simulink model "IEEE123bus_v2019b_Discrete_ZIPload"  (R2019b)
settings: Solver=ode4  StartTime=0.0  StopTime=5  FixedStep=Ts  MaxStep=1e-4  RelTol=1e-3
InitFcn:
  | a=1; % Loading Factor
  | Ts=50e-6;
  | % phase to sequence conversion of RXB matrices
  | c=1*exp(sqrt(-1)*(120*pi/180));
  | T=[1 1 1;1 c*c c;1 c c*c];
  | Tinv=1/3*[1 1 1;1 c c*c;1 c*c c];
  | 
  | % Simulation data for the IEEE 123 Node Test Feeder model
  | mi2km = 1.60934;%  miles to km conversion
  | ft2km = 0.0003048; % feet to km conversion
  | ms2F = 1*1e-6/(2*pi*60);% microsiemens to Farads conversion
  | 
  | %% Configuration 1
  | % Series Resitance and Reactance - ohm/mile
  | R_1 = [0.4576 0.1560 0.1535;0.1560 0.4666 0.1580;0.1535 0.1580 0.4615];
  | X_1 = [1.0780 0.5017 0.3849;0.5017 1.0482 0.4236;0.3849 0.4236 1.0651];
  | % charging susceptance - microsiemens/mile
  | B_1 = [5.6765 -1.8319 -0.6982;-1.8319 5.9809 -1.1645;-0.6982 -1.1645 5.3971];
  | 
  | R_1 = R_1/mi2km;
  | Rseq=Tinv*R_1*T;
  | R1_1=Rseq(2,2);R0_1=Rseq(1,1);
  | 
  | L_1 = (X_1/(2*pi*60))/mi2km;
  | Lseq=Tinv*L_1*T;
  | L1_1=Lseq(2,2);L0_1=Lseq(1,1);
  | 
  | C_1 =(B_1*ms2F)/mi2km;
  | Cseq=Tinv*C_1*T;
  | C1_1=Cseq(2,2);C0_1=Cseq(1,1);
  | %% Configuration 2 - series reactance - ohm/mile
  | R_2 = [0.4666 0.1580 0.1560;0.1580 0.4615 0.1535;0.1560 0.1535 0.4576];
  | X_2 = [1.0482 0.4236 0.5017;0.4236 1.0651 0.3849;0.5017 0.3849 1.0780];
  | % charging susceptance - microsiemens/mile
  | B_2 = [5.9809 -1.1645 -1.8319;-1.1645 5.3971 -0.6982;-1.8319 -0.6982 5.6765];
  | 
  | R_2 = R_2/mi2km;
  | Rseq=Tinv*R_2*T;
  | R1_2=Rseq(2,2);R0_2=Rseq(1,1);
  | 
  | L_2 = (X_2/(2*pi*60))/mi2km;
  | Lseq=Tinv*L_2*T;
  | L1_2=Lseq(2,2);L0_2=Lseq(1,1);
  | 
  | C_2 =(B_2*ms2F)/mi2km;
  | Cseq=Tinv*C_2*T;
  | C1_2=Cseq(2,2);C0_2=Cseq(1,1);
  | %% Configuration 3 - series reactance - ohm/mile
  | R_3 = [0.4615 0.1535 0.1580;0.1535 0.4576 0.1560;0.1580 0.1560 0.4666];
  | X_3 = [1.0651 0.3849 0.4236;0.3849 1.0780 0.5017;0.4236 0.5017 1.0482];
  | % charging susceptance - microsiemens/mile
  | B_3 = [5.3971 -0.6982 -1.1645;-0.6982 5.6765 -1.8319; -1.1645 -1.8319 5.9809];
  | 
  | R_3 = R_3/mi2km;
  | Rseq=Tinv*R_3*T;
  | R1_3=Rseq(2,2);R0_3=Rseq(1,1);
  | 
  | L_3 = (X_3/(2*pi*60))/mi2km;
  | Lseq=Tinv*L_3*T;
  | L1_3=Lseq(2,2);L0_3=Lseq(1,1);
  | ... (+157 lines)
undefined symbols (not defined in the file): D1, Delta, find_system
libraries: powerlib x971, powerlib_meascontrol x294
(part 3 of 14)

== system IEEE123bus_v2019b_Discrete_ZIPload/1 Y PQ ==
  "    1" : Gain  Gain=pi/180
  "    2" : Gain  Gain=pi/180
  "    3" : Gain  Gain=pi/180
  "    4" : Gain  Gain=1/sqrt(2)
  Clock : Clock
  Controlled Current Source : powerlib/Electrical Sources/Controlled Current Source  Initialize=off  Source_Type=AC  Amplitude=0  Phase=0  Frequency=0  Measurements=None
      settings: SourceProductName=Simscape Electrical
  Embedded MATLAB Function : MATLAB Function  TreatAsAtomicUnit=on
  Fourier : powerlib_meascontrol/Measurements/Fourier  Freq=60  n=1  InInit=[Vnom*sqrt(2) 0]  Ts=Ts
      settings: SourceProductName=Simscape Electrical
  Fourier1 : powerlib_meascontrol/Measurements/Fourier  Freq=60  n=1  InInit=[Vnom*sqrt(2) 0]  Ts=Ts
      settings: SourceProductName=Simscape Electrical
  Fourier2 : powerlib_meascontrol/Measurements/Fourier  Freq=60  n=1  InInit=[Vnom*sqrt(2) 0]  Ts=Ts
      settings: SourceProductName=Simscape Electrical
  Magnitude-Angle to Complex : MagnitudeAngleToComplex
  Memory1 : Memory
  Memory2 : Memory
  Rc+jXc1 : powerlib/Elements/Series RLC Branch  LConnTagsString=__new0  RConnTagsString=__new0  BranchType=R  Resistance=1e6  Inductance=1.6 / (120*pi) * 2  SetiL0=off  InitialCurrent=0  Capacitance=1e-6  Setx0=off  InitialVoltage=0  Measurements=None
      settings: SourceProductName=Simscape Electrical
  Sum : Sum  Inputs=|+-
  Voltage Measurement1 : powerlib/Measurements/Voltage Measurement  PhasorSimulation=off  OutputType=Complex  PSBequivalent=0
      settings: SourceProductName=Simscape Electrical
  " " : PMIOPort  Tag=PMCPort  Side=Left
  " 1" : PMIOPort  Tag=PMCPort  Port=2  Side=Right
  wires:
  Fourier/2 -> "    3"/1
  "    1"/1 -> Sum/1
  Voltage Measurement1/1 -> [v]
  [del] -> Embedded MATLAB Function/3(Ddel)
  Memory2/1 -> [del]
  Sum/1 -> Memory2/1
  "    2"/1 -> Sum/2
  [v] -> Fourier/1
  Fourier/1 -> "    4"/1
  Embedded MATLAB Function/1(Iinjinst) -> Memory1/1, Fourier1/1
  Fourier1/2 -> "    1"/1
  Memory1/1 -> Controlled Current Source/1, Fourier2/1
  Clock/1 -> Embedded MATLAB Function/2(clock)
  Magnitude-Angle to Complex/1 -> Embedded MATLAB Function/1(Vmeas)
  "    4"/1 -> Magnitude-Angle to Complex/1
  Fourier2/2 -> "    2"/1
  "    3"/1 -> Magnitude-Angle to Complex/2
  connections:
  Rc+jXc1/LConn1 -- Voltage Measurement1/LConn1 -- " "/RConn1 -- Controlled Current Source/LConn1
  Voltage Measurement1/LConn2 -- " 1"/RConn1 -- Controlled Current Source/RConn1 -- Rc+jXc1/RConn1

== system IEEE123bus_v2019b_Discrete_ZIPload/10 ==
  2 : powerlib/Measurements/Three-Phase V-I Measurement  VoltageMeasurement=phase-to-ground  SetLabelV=on  LabelV=V10  Vpu=off  VpuLL=off  CurrentMeasurement=no  SetLabelI=on  LabelI=I800  Ipu=off  Pbase=100e6  Vbase=24900  OutputType=Complex  PhasorSimulation=on  PSBequivalent=0
      settings: SourceProductName=Simscape Electrical
  Ground82 : powerlib/Elements/Ground  LConnTagsString=a
      settings: SourceProductName=Simscape Electrical
  Ground83 : powerlib/Elements/Ground  LConnTagsString=a
      settings: SourceProductName=Simscape Electrical
  a : PMIOPort  Side=Right
  A : PMIOPort  Port=2  Side=Left
  connections:
  A/RConn1 -- 2/LConn1
  a/RConn1 -- 2/RConn1
  2/LConn2 -- 2/LConn3 -- Ground83/LConn1
  2/RConn2 -- 2/RConn3 -- Ground82/LConn1

== system IEEE123bus_v2019b_Discrete_ZIPload/10 Y I ==
  "    1" : Gain  Gain=pi/180
  "    2" : Gain  Gain=pi/180
  "    3" : Gain  Gain=pi/180
  "    4" : Gain  Gain=1/sqrt(2)
  Clock : Clock
  Controlled Current Source : powerlib/Electrical Sources/Controlled Current Source  Initialize=off  Source_Type=AC  Amplitude=0  Phase=0  Frequency=0  Measurements=None
      settings: SourceProductName=Simscape Electrical
  Embedded MATLAB Function : MATLAB Function  TreatAsAtomicUnit=on
  Fourier : powerlib_meascontrol/Measurements/Fourier  Freq=60  n=1  InInit=[Vnom*sqrt(2) 0]  Ts=Ts
      settings: SourceProductName=Simscape Electrical
  Fourier1 : powerlib_meascontrol/Measurements/Fourier  Freq=60  n=1  InInit=[Vnom*sqrt(2) 0]  Ts=Ts
      settings: SourceProductName=Simscape Electrical
  Fourier2 : powerlib_meascontrol/Measurements/Fourier  Freq=60  n=1  InInit=[Vnom*sqrt(2) 0]  Ts=Ts
      settings: SourceProductName=Simscape Electrical
  Magnitude-Angle to Complex : MagnitudeAngleToComplex
  Memory1 : Memory
  Memory2 : Memory
  Rc+jXc1 : powerlib/Elements/Series RLC Branch  LConnTagsString=__new0  RConnTagsString=__new0  BranchType=R  Resistance=1e6  Inductance=1.6 / (120*pi) * 2  SetiL0=off  InitialCurrent=0  Capacitance=1e-6  Setx0=off  InitialVoltage=0  Measurements=None
      settings: SourceProductName=Simscape Electrical
  Sum : Sum  Inputs=|+-
  Voltage Measurement1 : powerlib/Measurements/Voltage Measurement  PhasorSimulation=off  OutputType=Complex  PSBequivalent=0
      settings: SourceProductName=Simscape Electrical
  " " : PMIOPort  Tag=PMCPort  Side=Left
  " 1" : PMIOPort  Tag=PMCPort  Port=2  Side=Right
  wires:
  Fourier/2 -> "    3"/1
  "    1"/1 -> Sum/1
  Voltage Measurement1/1 -> [v]
  [del] -> Embedded MATLAB Function/3(Ddel)
  Memory2/1 -> [del]
  Sum/1 -> Memory2/1
  "    2"/1 -> Sum/2
  [v] -> Fourier/1
  Fourier/1 -> "    4"/1
  Embedded MATLAB Function/1(Iinjinst) -> Memory1/1, Fourier1/1
  Fourier1/2 -> "    1"/1
  Memory1/1 -> Controlled Current Source/1, Fourier2/1
  Clock/1 -> Embedded MATLAB Function/2(clock)
  Magnitude-Angle to Complex/1 -> Embedded MATLAB Function/1(Vmeas)
  "    4"/1 -> Magnitude-Angle to Complex/1
  Fourier2/2 -> "    2"/1
  "    3"/1 -> Magnitude-Angle to Complex/2
  connections:
  Rc+jXc1/LConn1 -- Voltage Measurement1/LConn1 -- " "/RConn1 -- Controlled Current Source/LConn1
  Voltage Measurement1/LConn2 -- " 1"/RConn1 -- Controlled Current Source/RConn1 -- Rc+jXc1/RConn1

== system IEEE123bus_v2019b_Discrete_ZIPload/100 Y Z ==
  "    1" : Gain  Gain=pi/180
  "    2" : Gain  Gain=pi/180
  "    3" : Gain  Gain=pi/180
  "    4" : Gain  Gain=1/sqrt(2)
  Clock : Clock
  Controlled Current Source : powerlib/Electrical Sources/Controlled Current Source  Initialize=off  Source_Type=AC  Amplitude=0  Phase=0  Frequency=0  Measurements=None
      settings: SourceProductName=Simscape Electrical
  Embedded MATLAB Function : MATLAB Function  TreatAsAtomicUnit=on
  Fourier : powerlib_meascontrol/Measurements/Fourier  Freq=60  n=1  InInit=[Vnom*sqrt(2) 0]  Ts=Ts
      settings: SourceProductName=Simscape Electrical
  Fourier1 : powerlib_meascontrol/Measurements/Fourier  Freq=60  n=1  InInit=[Vnom*sqrt(2) 0]  Ts=Ts
      settings: SourceProductName=Simscape Electrical
  Fourier2 : powerlib_meascontrol/Measurements/Fourier  Freq=60  n=1  InInit=[Vnom*sqrt(2) 0]  Ts=Ts
      settings: SourceProductName=Simscape Electrical
  Magnitude-Angle to Complex : MagnitudeAngleToComplex
  Memory1 : Memory
  Memory2 : Memory
  Rc+jXc1 : powerlib/Elements/Series RLC Branch  LConnTagsString=__new0  RConnTagsString=__new0  BranchType=R  Resistance=1e6  Inductance=1.6 / (120*pi) * 2  SetiL0=off  InitialCurrent=0  Capacitance=1e-6  Setx0=off  InitialVoltage=0  Measurements=None
      settings: SourceProductName=Simscape Electrical
  Sum : Sum  Inputs=|+-
  Voltage Measurement1 : powerlib/Measurements/Voltage Measurement  PhasorSimulation=off  OutputType=Complex  PSBequivalent=0
      settings: SourceProductName=Simscape Electrical
  " " : PMIOPort  Tag=PMCPort  Side=Left
  " 1" : PMIOPort  Tag=PMCPort  Port=2  Side=Right
  wires:
  Fourier/2 -> "    3"/1
  "    1"/1 -> Sum/1
  Voltage Measurement1/1 -> [v]
  [del] -> Embedded MATLAB Function/3(Ddel)
  Memory2/1 -> [del]
  Sum/1 -> Memory2/1
  "    2"/1 -> Sum/2
  [v] -> Fourier/1
  Fourier/1 -> "    4"/1
  Embedded MATLAB Function/1(Iinjinst) -> Memory1/1, Fourier1/1
  Fourier1/2 -> "    1"/1
  Memory1/1 -> Controlled Current Source/1, Fourier2/1
  Clock/1 -> Embedded MATLAB Function/2(clock)
  Magnitude-Angle to Complex/1 -> Embedded MATLAB Function/1(Vmeas)
  "    4"/1 -> Magnitude-Angle to Complex/1
  Fourier2/2 -> "    2"/1
  "    3"/1 -> Magnitude-Angle to Complex/2
  connections:
  Rc+jXc1/LConn1 -- Voltage Measurement1/LConn1 -- " "/RConn1 -- Controlled Current Source/LConn1
  Voltage Measurement1/LConn2 -- " 1"/RConn1 -- Controlled Current Source/RConn1 -- Rc+jXc1/RConn1

== system IEEE123bus_v2019b_Discrete_ZIPload/102 ==
  2 : powerlib/Measurements/Three-Phase V-I Measurement  VoltageMeasurement=phase-to-ground  SetLabelV=on  LabelV=V102  Vpu=off  VpuLL=off  CurrentMeasurement=no  SetLabelI=on  LabelI=I800  Ipu=off  Pbase=100e6  Vbase=24900  OutputType=Complex  PhasorSimulation=on  PSBequivalent=0
      settings: SourceProductName=Simscape Electrical
  Ground82 : powerlib/Elements/Ground  LConnTagsString=a
      settings: SourceProductName=Simscape Electrical
  Ground83 : powerlib/Elements/Ground  LConnTagsString=a
      settings: SourceProductName=Simscape Electrical
  c : PMIOPort  Side=Right
  C : PMIOPort  Port=2  Side=Left
  connections:
  C/RConn1 -- 2/LConn3
  c/RConn1 -- 2/RConn3
  Ground82/LConn1 -- 2/RConn2 -- 2/RConn1
  Ground83/LConn1 -- 2/LConn2 -- 2/LConn1

== system IEEE123bus_v2019b_Discrete_ZIPload/102 Y PQ ==
  "    1" : Gain  Gain=pi/180
  "    2" : Gain  Gain=pi/180
  "    3" : Gain  Gain=pi/180
  "    4" : Gain  Gain=1/sqrt(2)
  Clock : Clock
  Controlled Current Source : powerlib/Electrical Sources/Controlled Current Source  Initialize=off  Source_Type=AC  Amplitude=0  Phase=0  Frequency=0  Measurements=None
      settings: SourceProductName=Simscape Electrical
  Embedded MATLAB Function : MATLAB Function  TreatAsAtomicUnit=on
  Fourier : powerlib_meascontrol/Measurements/Fourier  Freq=60  n=1  InInit=[Vnom*sqrt(2) 0]  Ts=Ts
      settings: SourceProductName=Simscape Electrical
  Fourier1 : powerlib_meascontrol/Measurements/Fourier  Freq=60  n=1  InInit=[Vnom*sqrt(2) 0]  Ts=Ts
      settings: SourceProductName=Simscape Electrical
  Fourier2 : powerlib_meascontrol/Measurements/Fourier  Freq=60  n=1  InInit=[Vnom*sqrt(2) 0]  Ts=Ts
      settings: SourceProductName=Simscape Electrical
  Magnitude-Angle to Complex : MagnitudeAngleToComplex
  Memory1 : Memory
  Memory2 : Memory
  Rc+jXc1 : powerlib/Elements/Series RLC Branch  LConnTagsString=__new0  RConnTagsString=__new0  BranchType=R  Resistance=1e6  Inductance=1.6 / (120*pi) * 2  SetiL0=off  InitialCurrent=0  Capacitance=1e-6  Setx0=off  InitialVoltage=0  Measurements=None
      settings: SourceProductName=Simscape Electrical
  Sum : Sum  Inputs=|+-
  Voltage Measurement1 : powerlib/Measurements/Voltage Measurement  PhasorSimulation=off  OutputType=Complex  PSBequivalent=0
      settings: SourceProductName=Simscape Electrical
  " " : PMIOPort  Tag=PMCPort  Side=Left
  " 1" : PMIOPort  Tag=PMCPort  Port=2  Side=Right
  wires:
  Fourier/2 -> "    3"/1
  "    1"/1 -> Sum/1
  Voltage Measurement1/1 -> [v]
  [del] -> Embedded MATLAB Function/3(Ddel)
  Memory2/1 -> [del]
  Sum/1 -> Memory2/1
  "    2"/1 -> Sum/2
  [v] -> Fourier/1
  Fourier/1 -> "    4"/1
  Embedded MATLAB Function/1(Iinjinst) -> Memory1/1, Fourier1/1
  Fourier1/2 -> "    1"/1
  Memory1/1 -> Controlled Current Source/1, Fourier2/1
  Clock/1 -> Embedded MATLAB Function/2(clock)
  Magnitude-Angle to Complex/1 -> Embedded MATLAB Function/1(Vmeas)
  "    4"/1 -> Magnitude-Angle to Complex/1
  Fourier2/2 -> "    2"/1
  "    3"/1 -> Magnitude-Angle to Complex/2
  connections:
  Rc+jXc1/LConn1 -- Voltage Measurement1/LConn1 -- " "/RConn1 -- Controlled Current Source/LConn1
  Voltage Measurement1/LConn2 -- " 1"/RConn1 -- Controlled Current Source/RConn1 -- Rc+jXc1/RConn1

== system IEEE123bus_v2019b_Discrete_ZIPload/103 ==
  2 : powerlib/Measurements/Three-Phase V-I Measurement  VoltageMeasurement=phase-to-ground  SetLabelV=on  LabelV=V103  Vpu=off  VpuLL=off  CurrentMeasurement=no  SetLabelI=on  LabelI=I800  Ipu=off  Pbase=100e6  Vbase=24900  OutputType=Complex  PhasorSimulation=on  PSBequivalent=0
      settings: SourceProductName=Simscape Electrical
  Ground82 : powerlib/Elements/Ground  LConnTagsString=a
      settings: SourceProductName=Simscape Electrical
  Ground83 : powerlib/Elements/Ground  LConnTagsString=a
      settings: SourceProductName=Simscape Electrical
  c : PMIOPort  Side=Right
  C : PMIOPort  Port=2  Side=Left
  connections:
  2/LConn1 -- 2/LConn2 -- Ground83/LConn1
  2/RConn1 -- 2/RConn2 -- Ground82/LConn1
  c/RConn1 -- 2/RConn3
  C/RConn1 -- 2/LConn3

== system IEEE123bus_v2019b_Discrete_ZIPload/103 Y PQ ==
  "    1" : Gain  Gain=pi/180
  "    2" : Gain  Gain=pi/180
  "    3" : Gain  Gain=pi/180
  "    4" : Gain  Gain=1/sqrt(2)
  Clock : Clock
  Controlled Current Source : powerlib/Electrical Sources/Controlled Current Source  Initialize=off  Source_Type=AC  Amplitude=0  Phase=0  Frequency=0  Measurements=None
      settings: SourceProductName=Simscape Electrical
  Embedded MATLAB Function : MATLAB Function  TreatAsAtomicUnit=on
  Fourier : powerlib_meascontrol/Measurements/Fourier  Freq=60  n=1  InInit=[Vnom*sqrt(2) 0]  Ts=Ts
      settings: SourceProductName=Simscape Electrical
  Fourier1 : powerlib_meascontrol/Measurements/Fourier  Freq=60  n=1  InInit=[Vnom*sqrt(2) 0]  Ts=Ts
      settings: SourceProductName=Simscape Electrical
  Fourier2 : powerlib_meascontrol/Measurements/Fourier  Freq=60  n=1  InInit=[Vnom*sqrt(2) 0]  Ts=Ts
      settings: SourceProductName=Simscape Electrical
  Magnitude-Angle to Complex : MagnitudeAngleToComplex
  Memory1 : Memory
  Memory2 : Memory
  Rc+jXc1 : powerlib/Elements/Series RLC Branch  LConnTagsString=__new0  RConnTagsString=__new0  BranchType=R  Resistance=1e6  Inductance=1.6 / (120*pi) * 2  SetiL0=off  InitialCurrent=0  Capacitance=1e-6  Setx0=off  InitialVoltage=0  Measurements=None
      settings: SourceProductName=Simscape Electrical
  Sum : Sum  Inputs=|+-
  Voltage Measurement1 : powerlib/Measurements/Voltage Measurement  PhasorSimulation=off  OutputType=Complex  PSBequivalent=0
      settings: SourceProductName=Simscape Electrical
  " " : PMIOPort  Tag=PMCPort  Side=Left
  " 1" : PMIOPort  Tag=PMCPort  Port=2  Side=Right
  wires:
  Fourier/2 -> "    3"/1
  "    1"/1 -> Sum/1
  Voltage Measurement1/1 -> [v]
  [del] -> Embedded MATLAB Function/3(Ddel)
  Memory2/1 -> [del]
  Sum/1 -> Memory2/1
  "    2"/1 -> Sum/2
  [v] -> Fourier/1
  Fourier/1 -> "    4"/1
  Embedded MATLAB Function/1(Iinjinst) -> Memory1/1, Fourier1/1
  Fourier1/2 -> "    1"/1
  Memory1/1 -> Controlled Current Source/1, Fourier2/1
  Clock/1 -> Embedded MATLAB Function/2(clock)
  Magnitude-Angle to Complex/1 -> Embedded MATLAB Function/1(Vmeas)
  "    4"/1 -> Magnitude-Angle to Complex/1
  Fourier2/2 -> "    2"/1
  "    3"/1 -> Magnitude-Angle to Complex/2
  connections:
  Rc+jXc1/LConn1 -- Voltage Measurement1/LConn1 -- " "/RConn1 -- Controlled Current Source/LConn1
  Voltage Measurement1/LConn2 -- " 1"/RConn1 -- Controlled Current Source/RConn1 -- Rc+jXc1/RConn1

== system IEEE123bus_v2019b_Discrete_ZIPload/104 ==
  2 : powerlib/Measurements/Three-Phase V-I Measurement  VoltageMeasurement=phase-to-ground  SetLabelV=on  LabelV=V104  Vpu=off  VpuLL=off  CurrentMeasurement=no  SetLabelI=on  LabelI=I800  Ipu=off  Pbase=100e6  Vbase=24900  OutputType=Complex  PhasorSimulation=on  PSBequivalent=0
      settings: SourceProductName=Simscape Electrical
  Ground82 : powerlib/Elements/Ground  LConnTagsString=a
      settings: SourceProductName=Simscape Electrical
  Ground83 : powerlib/Elements/Ground  LConnTagsString=a
      settings: SourceProductName=Simscape Electrical
  c : PMIOPort  Side=Right
  C : PMIOPort  Port=2  Side=Left
  connections:
  C/RConn1 -- 2/LConn3
  c/RConn1 -- 2/RConn3
  Ground82/LConn1 -- 2/RConn2 -- 2/RConn1
  Ground83/LConn1 -- 2/LConn2 -- 2/LConn1

== system IEEE123bus_v2019b_Discrete_ZIPload/104 Y PQ ==
  "    1" : Gain  Gain=pi/180
  "    2" : Gain  Gain=pi/180
  "    3" : Gain  Gain=pi/180
  "    4" : Gain  Gain=1/sqrt(2)
  Clock : Clock
  Controlled Current Source : powerlib/Electrical Sources/Controlled Current Source  Initialize=off  Source_Type=AC  Amplitude=0  Phase=0  Frequency=0  Measurements=None
      settings: SourceProductName=Simscape Electrical
  Embedded MATLAB Function : MATLAB Function  TreatAsAtomicUnit=on
  Fourier : powerlib_meascontrol/Measurements/Fourier  Freq=60  n=1  InInit=[Vnom*sqrt(2) 0]  Ts=Ts
      settings: SourceProductName=Simscape Electrical
  Fourier1 : powerlib_meascontrol/Measurements/Fourier  Freq=60  n=1  InInit=[Vnom*sqrt(2) 0]  Ts=Ts
      settings: SourceProductName=Simscape Electrical
  Fourier2 : powerlib_meascontrol/Measurements/Fourier  Freq=60  n=1  InInit=[Vnom*sqrt(2) 0]  Ts=Ts
      settings: SourceProductName=Simscape Electrical
  Magnitude-Angle to Complex : MagnitudeAngleToComplex
  Memory1 : Memory
  Memory2 : Memory
  Rc+jXc1 : powerlib/Elements/Series RLC Branch  LConnTagsString=__new0  RConnTagsString=__new0  BranchType=R  Resistance=1e6  Inductance=1.6 / (120*pi) * 2  SetiL0=off  InitialCurrent=0  Capacitance=1e-6  Setx0=off  InitialVoltage=0  Measurements=None
      settings: SourceProductName=Simscape Electrical
  Sum : Sum  Inputs=|+-
  Voltage Measurement1 : powerlib/Measurements/Voltage Measurement  PhasorSimulation=off  OutputType=Complex  PSBequivalent=0
      settings: SourceProductName=Simscape Electrical
  " " : PMIOPort  Tag=PMCPort  Side=Left
  " 1" : PMIOPort  Tag=PMCPort  Port=2  Side=Right
  wires:
  Fourier/2 -> "    3"/1
  "    1"/1 -> Sum/1
  Voltage Measurement1/1 -> [v]
  [del] -> Embedded MATLAB Function/3(Ddel)
  Memory2/1 -> [del]
  Sum/1 -> Memory2/1
  "    2"/1 -> Sum/2
  [v] -> Fourier/1
  Fourier/1 -> "    4"/1
  Embedded MATLAB Function/1(Iinjinst) -> Memory1/1, Fourier1/1
  Fourier1/2 -> "    1"/1
  Memory1/1 -> Controlled Current Source/1, Fourier2/1
  Clock/1 -> Embedded MATLAB Function/2(clock)
  Magnitude-Angle to Complex/1 -> Embedded MATLAB Function/1(Vmeas)
  "    4"/1 -> Magnitude-Angle to Complex/1
  Fourier2/2 -> "    2"/1
  "    3"/1 -> Magnitude-Angle to Complex/2
  connections:
  Rc+jXc1/LConn1 -- Voltage Measurement1/LConn1 -- " "/RConn1 -- Controlled Current Source/LConn1
  Voltage Measurement1/LConn2 -- " 1"/RConn1 -- Controlled Current Source/RConn1 -- Rc+jXc1/RConn1

== system IEEE123bus_v2019b_Discrete_ZIPload/106 ==
  2 : powerlib/Measurements/Three-Phase V-I Measurement  VoltageMeasurement=phase-to-ground  SetLabelV=on  LabelV=V106  Vpu=off  VpuLL=off  CurrentMeasurement=no  SetLabelI=on  LabelI=I800  Ipu=off  Pbase=100e6  Vbase=24900  OutputType=Complex  PhasorSimulation=on  PSBequivalent=0
      settings: SourceProductName=Simscape Electrical
  Ground82 : powerlib/Elements/Ground  LConnTagsString=a
      settings: SourceProductName=Simscape Electrical
  Ground83 : powerlib/Elements/Ground  LConnTagsString=a
      settings: SourceProductName=Simscape Electrical
  b : PMIOPort  Side=Right
  B : PMIOPort  Port=2  Side=Left
  connections:
  Ground82/LConn1 -- 2/RConn3 -- 2/RConn1
  Ground83/LConn1 -- 2/LConn3 -- 2/LConn1
  2/RConn2 -- b/RConn1
  2/LConn2 -- B/RConn1

== system IEEE123bus_v2019b_Discrete_ZIPload/106 Y PQ ==
  "    1" : Gain  Gain=pi/180
  "    2" : Gain  Gain=pi/180
  "    3" : Gain  Gain=pi/180
  "    4" : Gain  Gain=1/sqrt(2)
  Clock : Clock
  Controlled Current Source : powerlib/Electrical Sources/Controlled Current Source  Initialize=off  Source_Type=AC  Amplitude=0  Phase=0  Frequency=0  Measurements=None
      settings: SourceProductName=Simscape Electrical
  Embedded MATLAB Function : MATLAB Function  TreatAsAtomicUnit=on
  Fourier : powerlib_meascontrol/Measurements/Fourier  Freq=60  n=1  InInit=[Vnom*sqrt(2) 0]  Ts=Ts
      settings: SourceProductName=Simscape Electrical
  Fourier1 : powerlib_meascontrol/Measurements/Fourier  Freq=60  n=1  InInit=[Vnom*sqrt(2) 0]  Ts=Ts
      settings: SourceProductName=Simscape Electrical
  Fourier2 : powerlib_meascontrol/Measurements/Fourier  Freq=60  n=1  InInit=[Vnom*sqrt(2) 0]  Ts=Ts
      settings: SourceProductName=Simscape Electrical
  Magnitude-Angle to Complex : MagnitudeAngleToComplex
  Memory1 : Memory
  Memory2 : Memory
  Rc+jXc1 : powerlib/Elements/Series RLC Branch  LConnTagsString=__new0  RConnTagsString=__new0  BranchType=R  Resistance=1e6  Inductance=1.6 / (120*pi) * 2  SetiL0=off  InitialCurrent=0  Capacitance=1e-6  Setx0=off  InitialVoltage=0  Measurements=None
      settings: SourceProductName=Simscape Electrical
  Sum : Sum  Inputs=|+-
  Voltage Measurement1 : powerlib/Measurements/Voltage Measurement  PhasorSimulation=off  OutputType=Complex  PSBequivalent=0
      settings: SourceProductName=Simscape Electrical
  " " : PMIOPort  Tag=PMCPort  Side=Left
  " 1" : PMIOPort  Tag=PMCPort  Port=2  Side=Right
  wires:
  Fourier/2 -> "    3"/1
  "    1"/1 -> Sum/1
  Voltage Measurement1/1 -> [v]
  [del] -> Embedded MATLAB Function/3(Ddel)
  Memory2/1 -> [del]
  Sum/1 -> Memory2/1
  "    2"/1 -> Sum/2
  [v] -> Fourier/1
  Fourier/1 -> "    4"/1
  Embedded MATLAB Function/1(Iinjinst) -> Memory1/1, Fourier1/1
  Fourier1/2 -> "    1"/1
  Memory1/1 -> Controlled Current Source/1, Fourier2/1
  Clock/1 -> Embedded MATLAB Function/2(clock)
  Magnitude-Angle to Complex/1 -> Embedded MATLAB Function/1(Vmeas)
  "    4"/1 -> Magnitude-Angle to Complex/1
  Fourier2/2 -> "    2"/1
  "    3"/1 -> Magnitude-Angle to Complex/2
  connections:
  Rc+jXc1/LConn1 -- Voltage Measurement1/LConn1 -- " "/RConn1 -- Controlled Current Source/LConn1
  Voltage Measurement1/LConn2 -- " 1"/RConn1 -- Controlled Current Source/RConn1 -- Rc+jXc1/RConn1

== system IEEE123bus_v2019b_Discrete_ZIPload/107 ==
  2 : powerlib/Measurements/Three-Phase V-I Measurement  VoltageMeasurement=phase-to-ground  SetLabelV=on  LabelV=V107  Vpu=off  VpuLL=off  CurrentMeasurement=no  SetLabelI=on  LabelI=I800  Ipu=off  Pbase=100e6  Vbase=24900  OutputType=Complex  PhasorSimulation=on  PSBequivalent=0
      settings: SourceProductName=Simscape Electrical
  Ground82 : powerlib/Elements/Ground  LConnTagsString=a
      settings: SourceProductName=Simscape Electrical
  Ground83 : powerlib/Elements/Ground  LConnTagsString=a
      settings: SourceProductName=Simscape Electrical
  b : PMIOPort  Side=Right
  B : PMIOPort  Port=2  Side=Left
  connections:
  2/LConn2 -- B/RConn1
  2/RConn2 -- b/RConn1
  2/LConn1 -- 2/LConn3 -- Ground83/LConn1
  2/RConn1 -- 2/RConn3 -- Ground82/LConn1

== system IEEE123bus_v2019b_Discrete_ZIPload/107 Y PQ ==
  "    1" : Gain  Gain=pi/180
  "    2" : Gain  Gain=pi/180
  "    3" : Gain  Gain=pi/180
  "    4" : Gain  Gain=1/sqrt(2)
  Clock : Clock
  Controlled Current Source : powerlib/Electrical Sources/Controlled Current Source  Initialize=off  Source_Type=AC  Amplitude=0  Phase=0  Frequency=0  Measurements=None
      settings: SourceProductName=Simscape Electrical
  Embedded MATLAB Function : MATLAB Function  TreatAsAtomicUnit=on
  Fourier : powerlib_meascontrol/Measurements/Fourier  Freq=60  n=1  InInit=[Vnom*sqrt(2) 0]  Ts=Ts
      settings: SourceProductName=Simscape Electrical
  Fourier1 : powerlib_meascontrol/Measurements/Fourier  Freq=60  n=1  InInit=[Vnom*sqrt(2) 0]  Ts=Ts
      settings: SourceProductName=Simscape Electrical
  Fourier2 : powerlib_meascontrol/Measurements/Fourier  Freq=60  n=1  InInit=[Vnom*sqrt(2) 0]  Ts=Ts
      settings: SourceProductName=Simscape Electrical
  Magnitude-Angle to Complex : MagnitudeAngleToComplex
  Memory1 : Memory
  Memory2 : Memory
  Rc+jXc1 : powerlib/Elements/Series RLC Branch  LConnTagsString=__new0  RConnTagsString=__new0  BranchType=R  Resistance=1e6  Inductance=1.6 / (120*pi) * 2  SetiL0=off  InitialCurrent=0  Capacitance=1e-6  Setx0=off  InitialVoltage=0  Measurements=None
      settings: SourceProductName=Simscape Electrical
  Sum : Sum  Inputs=|+-
  Voltage Measurement1 : powerlib/Measurements/Voltage Measurement  PhasorSimulation=off  OutputType=Complex  PSBequivalent=0
      settings: SourceProductName=Simscape Electrical
  " " : PMIOPort  Tag=PMCPort  Side=Left
  " 1" : PMIOPort  Tag=PMCPort  Port=2  Side=Right
  wires:
  Fourier/2 -> "    3"/1
  "    1"/1 -> Sum/1
  Voltage Measurement1/1 -> [v]
  [del] -> Embedded MATLAB Function/3(Ddel)
  Memory2/1 -> [del]
  Sum/1 -> Memory2/1
  "    2"/1 -> Sum/2
  [v] -> Fourier/1
  Fourier/1 -> "    4"/1
  Embedded MATLAB Function/1(Iinjinst) -> Memory1/1, Fourier1/1
  Fourier1/2 -> "    1"/1
  Memory1/1 -> Controlled Current Source/1, Fourier2/1
  Clock/1 -> Embedded MATLAB Function/2(clock)
  Magnitude-Angle to Complex/1 -> Embedded MATLAB Function/1(Vmeas)
  "    4"/1 -> Magnitude-Angle to Complex/1
  Fourier2/2 -> "    2"/1
  "    3"/1 -> Magnitude-Angle to Complex/2
  connections:
  Rc+jXc1/LConn1 -- Voltage Measurement1/LConn1 -- " "/RConn1 -- Controlled Current Source/LConn1
  Voltage Measurement1/LConn2 -- " 1"/RConn1 -- Controlled Current Source/RConn1 -- Rc+jXc1/RConn1

== system IEEE123bus_v2019b_Discrete_ZIPload/109 ==
  2 : powerlib/Measurements/Three-Phase V-I Measurement  VoltageMeasurement=phase-to-ground  SetLabelV=on  LabelV=V109  Vpu=off  VpuLL=off  CurrentMeasurement=no  SetLabelI=on  LabelI=I800  Ipu=off  Pbase=100e6  Vbase=24900  OutputType=Complex  PhasorSimulation=on  PSBequivalent=0
      settings: SourceProductName=Simscape Electrical
  Ground82 : powerlib/Elements/Ground  LConnTagsString=a
      settings: SourceProductName=Simscape Electrical
  Ground83 : powerlib/Elements/Ground  LConnTagsString=a
      settings: SourceProductName=Simscape Electrical
  a : PMIOPort  Side=Right
  A : PMIOPort  Port=2  Side=Left
  connections:
  2/RConn3 -- 2/RConn2 -- Ground82/LConn1
  2/LConn3 -- 2/LConn2 -- Ground83/LConn1
  a/RConn1 -- 2/RConn1
  A/RConn1 -- 2/LConn1

== system IEEE123bus_v2019b_Discrete_ZIPload/109 Y PQ ==
  "    1" : Gain  Gain=pi/180
  "    2" : Gain  Gain=pi/180
  "    3" : Gain  Gain=pi/180
  "    4" : Gain  Gain=1/sqrt(2)
  Clock : Clock
  Controlled Current Source : powerlib/Electrical Sources/Controlled Current Source  Initialize=off  Source_Type=AC  Amplitude=0  Phase=0  Frequency=0  Measurements=None
      settings: SourceProductName=Simscape Electrical
  Embedded MATLAB Function : MATLAB Function  TreatAsAtomicUnit=on
  Fourier : powerlib_meascontrol/Measurements/Fourier  Freq=60  n=1  InInit=[Vnom*sqrt(2) 0]  Ts=Ts
      settings: SourceProductName=Simscape Electrical
  Fourier1 : powerlib_meascontrol/Measurements/Fourier  Freq=60  n=1  InInit=[Vnom*sqrt(2) 0]  Ts=Ts
      settings: SourceProductName=Simscape Electrical
  Fourier2 : powerlib_meascontrol/Measurements/Fourier  Freq=60  n=1  InInit=[Vnom*sqrt(2) 0]  Ts=Ts
      settings: SourceProductName=Simscape Electrical
  Magnitude-Angle to Complex : MagnitudeAngleToComplex
  Memory1 : Memory
  Memory2 : Memory
  Rc+jXc1 : powerlib/Elements/Series RLC Branch  LConnTagsString=__new0  RConnTagsString=__new0  BranchType=R  Resistance=1e6  Inductance=1.6 / (120*pi) * 2  SetiL0=off  InitialCurrent=0  Capacitance=1e-6  Setx0=off  InitialVoltage=0  Measurements=None
      settings: SourceProductName=Simscape Electrical
  Sum : Sum  Inputs=|+-
  Voltage Measurement1 : powerlib/Measurements/Voltage Measurement  PhasorSimulation=off  OutputType=Complex  PSBequivalent=0
      settings: SourceProductName=Simscape Electrical
  " " : PMIOPort  Tag=PMCPort  Side=Left
  " 1" : PMIOPort  Tag=PMCPort  Port=2  Side=Right
  wires:
  Fourier/2 -> "    3"/1
  "    1"/1 -> Sum/1
  Voltage Measurement1/1 -> [v]
  [del] -> Embedded MATLAB Function/3(Ddel)
  Memory2/1 -> [del]
  Sum/1 -> Memory2/1
  "    2"/1 -> Sum/2
  [v] -> Fourier/1
  Fourier/1 -> "    4"/1
  Embedded MATLAB Function/1(Iinjinst) -> Memory1/1, Fourier1/1
  Fourier1/2 -> "    1"/1
  Memory1/1 -> Controlled Current Source/1, Fourier2/1
  Clock/1 -> Embedded MATLAB Function/2(clock)
  Magnitude-Angle to Complex/1 -> Embedded MATLAB Function/1(Vmeas)
  "    4"/1 -> Magnitude-Angle to Complex/1
  Fourier2/2 -> "    2"/1
  "    3"/1 -> Magnitude-Angle to Complex/2
  connections:
  Rc+jXc1/LConn1 -- Voltage Measurement1/LConn1 -- " "/RConn1 -- Controlled Current Source/LConn1
  Voltage Measurement1/LConn2 -- " 1"/RConn1 -- Controlled Current Source/RConn1 -- Rc+jXc1/RConn1

== system IEEE123bus_v2019b_Discrete_ZIPload/11 ==
  2 : powerlib/Measurements/Three-Phase V-I Measurement  VoltageMeasurement=phase-to-ground  SetLabelV=on  LabelV=V11  Vpu=off  VpuLL=off  CurrentMeasurement=no  SetLabelI=on  LabelI=I800  Ipu=off  Pbase=100e6  Vbase=24900  OutputType=Complex  PhasorSimulation=on  PSBequivalent=0
      settings: SourceProductName=Simscape Electrical
  Ground82 : powerlib/Elements/Ground  LConnTagsString=a
      settings: SourceProductName=Simscape Electrical
  Ground83 : powerlib/Elements/Ground  LConnTagsString=a
      settings: SourceProductName=Simscape Electrical
  a : PMIOPort  Side=Right
  A : PMIOPort  Port=2  Side=Left
  connections:
  A/RConn1 -- 2/LConn1
  a/RConn1 -- 2/RConn1
  2/LConn2 -- 2/LConn3 -- Ground83/LConn1
  2/RConn2 -- 2/RConn3 -- Ground82/LConn1

== system IEEE123bus_v2019b_Discrete_ZIPload/11 Y Z ==
  "    1" : Gain  Gain=pi/180
  "    2" : Gain  Gain=pi/180
  "    3" : Gain  Gain=pi/180
  "    4" : Gain  Gain=1/sqrt(2)
  Clock : Clock
  Controlled Current Source : powerlib/Electrical Sources/Controlled Current Source  Initialize=off  Source_Type=AC  Amplitude=0  Phase=0  Frequency=0  Measurements=None
      settings: SourceProductName=Simscape Electrical
  Embedded MATLAB Function : MATLAB Function  TreatAsAtomicUnit=on
  Fourier : powerlib_meascontrol/Measurements/Fourier  Freq=60  n=1  InInit=[Vnom*sqrt(2) 0]  Ts=Ts
      settings: SourceProductName=Simscape Electrical
  Fourier1 : powerlib_meascontrol/Measurements/Fourier  Freq=60  n=1  InInit=[Vnom*sqrt(2) 0]  Ts=Ts
      settings: SourceProductName=Simscape Electrical
  Fourier2 : powerlib_meascontrol/Measurements/Fourier  Freq=60  n=1  InInit=[Vnom*sqrt(2) 0]  Ts=Ts
      settings: SourceProductName=Simscape Electrical
  Magnitude-Angle to Complex : MagnitudeAngleToComplex
  Memory1 : Memory
  Memory2 : Memory
  Rc+jXc1 : powerlib/Elements/Series RLC Branch  LConnTagsString=__new0  RConnTagsString=__new0  BranchType=R  Resistance=1e6  Inductance=1.6 / (120*pi) * 2  SetiL0=off  InitialCurrent=0  Capacitance=1e-6  Setx0=off  InitialVoltage=0  Measurements=None
      settings: SourceProductName=Simscape Electrical
  Sum : Sum  Inputs=|+-
  Voltage Measurement1 : powerlib/Measurements/Voltage Measurement  PhasorSimulation=off  OutputType=Complex  PSBequivalent=0
      settings: SourceProductName=Simscape Electrical
  " " : PMIOPort  Tag=PMCPort  Side=Left
  " 1" : PMIOPort  Tag=PMCPort  Port=2  Side=Right
  wires:
  Fourier/2 -> "    3"/1
  "    1"/1 -> Sum/1
  Voltage Measurement1/1 -> [v]
  [del] -> Embedded MATLAB Function/3(Ddel)
  Memory2/1 -> [del]
  Sum/1 -> Memory2/1
  "    2"/1 -> Sum/2
  [v] -> Fourier/1
  Fourier/1 -> "    4"/1
  Embedded MATLAB Function/1(Iinjinst) -> Memory1/1, Fourier1/1
  Fourier1/2 -> "    1"/1
  Memory1/1 -> Controlled Current Source/1, Fourier2/1
  Clock/1 -> Embedded MATLAB Function/2(clock)
  Magnitude-Angle to Complex/1 -> Embedded MATLAB Function/1(Vmeas)
  "    4"/1 -> Magnitude-Angle to Complex/1
  Fourier2/2 -> "    2"/1
  "    3"/1 -> Magnitude-Angle to Complex/2
  connections:
  Rc+jXc1/LConn1 -- Voltage Measurement1/LConn1 -- " "/RConn1 -- Controlled Current Source/LConn1
  Voltage Measurement1/LConn2 -- " 1"/RConn1 -- Controlled Current Source/RConn1 -- Rc+jXc1/RConn1

== system IEEE123bus_v2019b_Discrete_ZIPload/110 ==
  2 : powerlib/Measurements/Three-Phase V-I Measurement  VoltageMeasurement=phase-to-ground  SetLabelV=on  LabelV=V110  Vpu=off  VpuLL=off  CurrentMeasurement=no  SetLabelI=on  LabelI=I800  Ipu=off  Pbase=100e6  Vbase=24900  OutputType=Complex  PhasorSimulation=on  PSBequivalent=0
      settings: SourceProductName=Simscape Electrical
  Ground82 : powerlib/Elements/Ground  LConnTagsString=a
      settings: SourceProductName=Simscape Electrical
  Ground83 : powerlib/Elements/Ground  LConnTagsString=a
      settings: SourceProductName=Simscape Electrical
  a : PMIOPort  Side=Right
  A : PMIOPort  Port=2  Side=Left
  connections:
  A/RConn1 -- 2/LConn1
  a/RConn1 -- 2/RConn1
  Ground83/LConn1 -- 2/LConn2 -- 2/LConn3
  Ground82/LConn1 -- 2/RConn2 -- 2/RConn3

== system IEEE123bus_v2019b_Discrete_ZIPload/111 ==
  2 : powerlib/Measurements/Three-Phase V-I Measurement  VoltageMeasurement=phase-to-ground  SetLabelV=on  LabelV=V111  Vpu=off  VpuLL=off  CurrentMeasurement=no  SetLabelI=on  LabelI=I800  Ipu=off  Pbase=100e6  Vbase=24900  OutputType=Complex  PhasorSimulation=on  PSBequivalent=0
      settings: SourceProductName=Simscape Electrical
  Ground82 : powerlib/Elements/Ground  LConnTagsString=a
      settings: SourceProductName=Simscape Electrical
  Ground83 : powerlib/Elements/Ground  LConnTagsString=a
      settings: SourceProductName=Simscape Electrical
  a : PMIOPort  Side=Right
  A : PMIOPort  Port=2  Side=Left
  connections:
  2/RConn3 -- 2/RConn2 -- Ground82/LConn1
  2/LConn3 -- 2/LConn2 -- Ground83/LConn1
  a/RConn1 -- 2/RConn1
  A/RConn1 -- 2/LConn1

== system IEEE123bus_v2019b_Discrete_ZIPload/111 Y PQ ==
  "    1" : Gain  Gain=pi/180
  "    2" : Gain  Gain=pi/180
  "    3" : Gain  Gain=pi/180
  "    4" : Gain  Gain=1/sqrt(2)
  Clock : Clock
  Controlled Current Source : powerlib/Electrical Sources/Controlled Current Source  Initialize=off  Source_Type=AC  Amplitude=0  Phase=0  Frequency=0  Measurements=None
      settings: SourceProductName=Simscape Electrical
  Embedded MATLAB Function : MATLAB Function  TreatAsAtomicUnit=on
  Fourier : powerlib_meascontrol/Measurements/Fourier  Freq=60  n=1  InInit=[Vnom*sqrt(2) 0]  Ts=Ts
      settings: SourceProductName=Simscape Electrical
  Fourier1 : powerlib_meascontrol/Measurements/Fourier  Freq=60  n=1  InInit=[Vnom*sqrt(2) 0]  Ts=Ts
      settings: SourceProductName=Simscape Electrical
  Fourier2 : powerlib_meascontrol/Measurements/Fourier  Freq=60  n=1  InInit=[Vnom*sqrt(2) 0]  Ts=Ts
      settings: SourceProductName=Simscape Electrical
  Magnitude-Angle to Complex : MagnitudeAngleToComplex
  Memory1 : Memory
  Memory2 : Memory
  Rc+jXc1 : powerlib/Elements/Series RLC Branch  LConnTagsString=__new0  RConnTagsString=__new0  BranchType=R  Resistance=1e6  Inductance=1.6 / (120*pi) * 2  SetiL0=off  InitialCurrent=0  Capacitance=1e-6  Setx0=off  InitialVoltage=0  Measurements=None
      settings: SourceProductName=Simscape Electrical
  Sum : Sum  Inputs=|+-
  Voltage Measurement1 : powerlib/Measurements/Voltage Measurement  PhasorSimulation=off  OutputType=Complex  PSBequivalent=0
      settings: SourceProductName=Simscape Electrical
  " " : PMIOPort  Tag=PMCPort  Side=Left
  " 1" : PMIOPort  Tag=PMCPort  Port=2  Side=Right
  wires:
  Fourier/2 -> "    3"/1
  "    1"/1 -> Sum/1
  Voltage Measurement1/1 -> [v]
  [del] -> Embedded MATLAB Function/3(Ddel)
  Memory2/1 -> [del]
  Sum/1 -> Memory2/1
  "    2"/1 -> Sum/2
  [v] -> Fourier/1
  Fourier/1 -> "    4"/1
  Embedded MATLAB Function/1(Iinjinst) -> Memory1/1, Fourier1/1
  Fourier1/2 -> "    1"/1
  Memory1/1 -> Controlled Current Source/1, Fourier2/1
  Clock/1 -> Embedded MATLAB Function/2(clock)
  Magnitude-Angle to Complex/1 -> Embedded MATLAB Function/1(Vmeas)
  "    4"/1 -> Magnitude-Angle to Complex/1
  Fourier2/2 -> "    2"/1
  "    3"/1 -> Magnitude-Angle to Complex/2
  connections:
  Rc+jXc1/LConn1 -- Voltage Measurement1/LConn1 -- " "/RConn1 -- Controlled Current Source/LConn1
  Voltage Measurement1/LConn2 -- " 1"/RConn1 -- Controlled Current Source/RConn1 -- Rc+jXc1/RConn1

== system IEEE123bus_v2019b_Discrete_ZIPload/112 ==
  2 : powerlib/Measurements/Three-Phase V-I Measurement  VoltageMeasurement=phase-to-ground  SetLabelV=on  LabelV=V112  Vpu=off  VpuLL=off  CurrentMeasurement=no  SetLabelI=on  LabelI=I800  Ipu=off  Pbase=100e6  Vbase=24900  OutputType=Complex  PhasorSimulation=on  PSBequivalent=0
      settings: SourceProductName=Simscape Electrical
  Ground82 : powerlib/Elements/Ground  LConnTagsString=a
      settings: SourceProductName=Simscape Electrical
  Ground83 : powerlib/Elements/Ground  LConnTagsString=a
      settings: SourceProductName=Simscape Electrical
  a : PMIOPort  Side=Right
  A : PMIOPort  Port=2  Side=Left
  connections:
  2/RConn3 -- 2/RConn2 -- Ground82/LConn1
  2/LConn3 -- 2/LConn2 -- Ground83/LConn1
  a/RConn1 -- 2/RConn1
  A/RConn1 -- 2/LConn1

== system IEEE123bus_v2019b_Discrete_ZIPload/112 Y I ==
  "    1" : Gain  Gain=pi/180
  "    2" : Gain  Gain=pi/180
  "    3" : Gain  Gain=pi/180
  "    4" : Gain  Gain=1/sqrt(2)
  Clock : Clock
  Controlled Current Source : powerlib/Electrical Sources/Controlled Current Source  Initialize=off  Source_Type=AC  Amplitude=0  Phase=0  Frequency=0  Measurements=None
      settings: SourceProductName=Simscape Electrical
  Embedded MATLAB Function : MATLAB Function  TreatAsAtomicUnit=on
  Fourier : powerlib_meascontrol/Measurements/Fourier  Freq=60  n=1  InInit=[Vnom*sqrt(2) 0]  Ts=Ts
      settings: SourceProductName=Simscape Electrical
  Fourier1 : powerlib_meascontrol/Measurements/Fourier  Freq=60  n=1  InInit=[Vnom*sqrt(2) 0]  Ts=Ts
      settings: SourceProductName=Simscape Electrical
  Fourier2 : powerlib_meascontrol/Measurements/Fourier  Freq=60  n=1  InInit=[Vnom*sqrt(2) 0]  Ts=Ts
      settings: SourceProductName=Simscape Electrical
  Magnitude-Angle to Complex : MagnitudeAngleToComplex
  Memory1 : Memory
  Memory2 : Memory
  Rc+jXc1 : powerlib/Elements/Series RLC Branch  LConnTagsString=__new0  RConnTagsString=__new0  BranchType=R  Resistance=1e6  Inductance=1.6 / (120*pi) * 2  SetiL0=off  InitialCurrent=0  Capacitance=1e-6  Setx0=off  InitialVoltage=0  Measurements=None
      settings: SourceProductName=Simscape Electrical
  Sum : Sum  Inputs=|+-
  Voltage Measurement1 : powerlib/Measurements/Voltage Measurement  PhasorSimulation=off  OutputType=Complex  PSBequivalent=0
      settings: SourceProductName=Simscape Electrical
  " " : PMIOPort  Tag=PMCPort  Side=Left
  " 1" : PMIOPort  Tag=PMCPort  Port=2  Side=Right
  wires:
  Fourier/2 -> "    3"/1
  "    1"/1 -> Sum/1
  Voltage Measurement1/1 -> [v]
  [del] -> Embedded MATLAB Function/3(Ddel)
  Memory2/1 -> [del]
  Sum/1 -> Memory2/1
  "    2"/1 -> Sum/2
  [v] -> Fourier/1
  Fourier/1 -> "    4"/1
  Embedded MATLAB Function/1(Iinjinst) -> Memory1/1, Fourier1/1
  Fourier1/2 -> "    1"/1
  Memory1/1 -> Controlled Current Source/1, Fourier2/1
  Clock/1 -> Embedded MATLAB Function/2(clock)
  Magnitude-Angle to Complex/1 -> Embedded MATLAB Function/1(Vmeas)
  "    4"/1 -> Magnitude-Angle to Complex/1
  Fourier2/2 -> "    2"/1
  "    3"/1 -> Magnitude-Angle to Complex/2
  connections:
  Rc+jXc1/LConn1 -- Voltage Measurement1/LConn1 -- " "/RConn1 -- Controlled Current Source/LConn1
  Voltage Measurement1/LConn2 -- " 1"/RConn1 -- Controlled Current Source/RConn1 -- Rc+jXc1/RConn1

== system IEEE123bus_v2019b_Discrete_ZIPload/113 ==
  2 : powerlib/Measurements/Three-Phase V-I Measurement  VoltageMeasurement=phase-to-ground  SetLabelV=on  LabelV=V113  Vpu=off  VpuLL=off  CurrentMeasurement=no  SetLabelI=on  LabelI=I800  Ipu=off  Pbase=100e6  Vbase=24900  OutputType=Complex  PhasorSimulation=on  PSBequivalent=0
      settings: SourceProductName=Simscape Electrical
  Ground82 : powerlib/Elements/Ground  LConnTagsString=a
      settings: SourceProductName=Simscape Electrical
  Ground83 : powerlib/Elements/Ground  LConnTagsString=a
      settings: SourceProductName=Simscape Electrical
  a : PMIOPort  Side=Right
  A : PMIOPort  Port=2  Side=Left
  connections:
  A/RConn1 -- 2/LConn1
  a/RConn1 -- 2/RConn1
  Ground83/LConn1 -- 2/LConn2 -- 2/LConn3
  Ground82/LConn1 -- 2/RConn2 -- 2/RConn3

== system IEEE123bus_v2019b_Discrete_ZIPload/113 Y Z ==
  "    1" : Gain  Gain=pi/180
  "    2" : Gain  Gain=pi/180
  "    3" : Gain  Gain=pi/180
  "    4" : Gain  Gain=1/sqrt(2)
  Clock : Clock
  Controlled Current Source : powerlib/Electrical Sources/Controlled Current Source  Initialize=off  Source_Type=AC  Amplitude=0  Phase=0  Frequency=0  Measurements=None
      settings: SourceProductName=Simscape Electrical
  Embedded MATLAB Function : MATLAB Function  TreatAsAtomicUnit=on
  Fourier : powerlib_meascontrol/Measurements/Fourier  Freq=60  n=1  InInit=[Vnom*sqrt(2) 0]  Ts=Ts
      settings: SourceProductName=Simscape Electrical
  Fourier1 : powerlib_meascontrol/Measurements/Fourier  Freq=60  n=1  InInit=[Vnom*sqrt(2) 0]  Ts=Ts
      settings: SourceProductName=Simscape Electrical
  Fourier2 : powerlib_meascontrol/Measurements/Fourier  Freq=60  n=1  InInit=[Vnom*sqrt(2) 0]  Ts=Ts
      settings: SourceProductName=Simscape Electrical
  Magnitude-Angle to Complex : MagnitudeAngleToComplex
  Memory1 : Memory
  Memory2 : Memory
  Rc+jXc1 : powerlib/Elements/Series RLC Branch  LConnTagsString=__new0  RConnTagsString=__new0  BranchType=R  Resistance=1e6  Inductance=1.6 / (120*pi) * 2  SetiL0=off  InitialCurrent=0  Capacitance=1e-6  Setx0=off  InitialVoltage=0  Measurements=None
      settings: SourceProductName=Simscape Electrical
  Sum : Sum  Inputs=|+-
  Voltage Measurement1 : powerlib/Measurements/Voltage Measurement  PhasorSimulation=off  OutputType=Complex  PSBequivalent=0
      settings: SourceProductName=Simscape Electrical
  " " : PMIOPort  Tag=PMCPort  Side=Left
  " 1" : PMIOPort  Tag=PMCPort  Port=2  Side=Right
  wires:
  Fourier/2 -> "    3"/1
  "    1"/1 -> Sum/1
  Voltage Measurement1/1 -> [v]
  [del] -> Embedded MATLAB Function/3(Ddel)
  Memory2/1 -> [del]
  Sum/1 -> Memory2/1
  "    2"/1 -> Sum/2
  [v] -> Fourier/1
  Fourier/1 -> "    4"/1
  Embedded MATLAB Function/1(Iinjinst) -> Memory1/1, Fourier1/1
  Fourier1/2 -> "    1"/1
  Memory1/1 -> Controlled Current Source/1, Fourier2/1
  Clock/1 -> Embedded MATLAB Function/2(clock)
  Magnitude-Angle to Complex/1 -> Embedded MATLAB Function/1(Vmeas)
  "    4"/1 -> Magnitude-Angle to Complex/1
  Fourier2/2 -> "    2"/1
  "    3"/1 -> Magnitude-Angle to Complex/2
  connections:
  Rc+jXc1/LConn1 -- Voltage Measurement1/LConn1 -- " "/RConn1 -- Controlled Current Source/LConn1
  Voltage Measurement1/LConn2 -- " 1"/RConn1 -- Controlled Current Source/RConn1 -- Rc+jXc1/RConn1

== system IEEE123bus_v2019b_Discrete_ZIPload/114 ==
  2 : powerlib/Measurements/Three-Phase V-I Measurement  VoltageMeasurement=phase-to-ground  SetLabelV=on  LabelV=V114  Vpu=off  VpuLL=off  CurrentMeasurement=no  SetLabelI=on  LabelI=I800  Ipu=off  Pbase=100e6  Vbase=24900  OutputType=Complex  PhasorSimulation=on  PSBequivalent=0
      settings: SourceProductName=Simscape Electrical
  Ground82 : powerlib/Elements/Ground  LConnTagsString=a
      settings: SourceProductName=Simscape Electrical
  Ground83 : powerlib/Elements/Ground  LConnTagsString=a
      settings: SourceProductName=Simscape Electrical
  a : PMIOPort  Side=Right
  A : PMIOPort  Port=2  Side=Left
  connections:
  2/RConn3 -- 2/RConn2 -- Ground82/LConn1
  2/LConn3 -- 2/LConn2 -- Ground83/LConn1
  a/RConn1 -- 2/RConn1
  A/RConn1 -- 2/LConn1

== system IEEE123bus_v2019b_Discrete_ZIPload/114 Y PQ ==
  "    1" : Gain  Gain=pi/180
  "    2" : Gain  Gain=pi/180
  "    3" : Gain  Gain=pi/180
  "    4" : Gain  Gain=1/sqrt(2)
  Clock : Clock
  Controlled Current Source : powerlib/Electrical Sources/Controlled Current Source  Initialize=off  Source_Type=AC  Amplitude=0  Phase=0  Frequency=0  Measurements=None
      settings: SourceProductName=Simscape Electrical
  Embedded MATLAB Function : MATLAB Function  TreatAsAtomicUnit=on
  Fourier : powerlib_meascontrol/Measurements/Fourier  Freq=60  n=1  InInit=[Vnom*sqrt(2) 0]  Ts=Ts
      settings: SourceProductName=Simscape Electrical
  Fourier1 : powerlib_meascontrol/Measurements/Fourier  Freq=60  n=1  InInit=[Vnom*sqrt(2) 0]  Ts=Ts
      settings: SourceProductName=Simscape Electrical
  Fourier2 : powerlib_meascontrol/Measurements/Fourier  Freq=60  n=1  InInit=[Vnom*sqrt(2) 0]  Ts=Ts
      settings: SourceProductName=Simscape Electrical
  Magnitude-Angle to Complex : MagnitudeAngleToComplex
  Memory1 : Memory
  Memory2 : Memory
  Rc+jXc1 : powerlib/Elements/Series RLC Branch  LConnTagsString=__new0  RConnTagsString=__new0  BranchType=R  Resistance=1e6  Inductance=1.6 / (120*pi) * 2  SetiL0=off  InitialCurrent=0  Capacitance=1e-6  Setx0=off  InitialVoltage=0  Measurements=None
      settings: SourceProductName=Simscape Electrical
  Sum : Sum  Inputs=|+-
  Voltage Measurement1 : powerlib/Measurements/Voltage Measurement  PhasorSimulation=off  OutputType=Complex  PSBequivalent=0
      settings: SourceProductName=Simscape Electrical
  " " : PMIOPort  Tag=PMCPort  Side=Left
  " 1" : PMIOPort  Tag=PMCPort  Port=2  Side=Right
  wires:
  Fourier/2 -> "    3"/1
  "    1"/1 -> Sum/1
  Voltage Measurement1/1 -> [v]
  [del] -> Embedded MATLAB Function/3(Ddel)
  Memory2/1 -> [del]
  Sum/1 -> Memory2/1
  "    2"/1 -> Sum/2
  [v] -> Fourier/1
  Fourier/1 -> "    4"/1
  Embedded MATLAB Function/1(Iinjinst) -> Memory1/1, Fourier1/1
  Fourier1/2 -> "    1"/1
  Memory1/1 -> Controlled Current Source/1, Fourier2/1
  Clock/1 -> Embedded MATLAB Function/2(clock)
  Magnitude-Angle to Complex/1 -> Embedded MATLAB Function/1(Vmeas)
  "    4"/1 -> Magnitude-Angle to Complex/1
  Fourier2/2 -> "    2"/1
  "    3"/1 -> Magnitude-Angle to Complex/2
  connections:
  Rc+jXc1/LConn1 -- Voltage Measurement1/LConn1 -- " "/RConn1 -- Controlled Current Source/LConn1
  Voltage Measurement1/LConn2 -- " 1"/RConn1 -- Controlled Current Source/RConn1 -- Rc+jXc1/RConn1

== system IEEE123bus_v2019b_Discrete_ZIPload/12 ==
  2 : powerlib/Measurements/Three-Phase V-I Measurement  VoltageMeasurement=phase-to-ground  SetLabelV=on  LabelV=V12  Vpu=off  VpuLL=off  CurrentMeasurement=no  SetLabelI=on  LabelI=I800  Ipu=off  Pbase=100e6  Vbase=24900  OutputType=Complex  PhasorSimulation=on  PSBequivalent=0
      settings: SourceProductName=Simscape Electrical
  Ground82 : powerlib/Elements/Ground  LConnTagsString=a
      settings: SourceProductName=Simscape Electrical
  Ground83 : powerlib/Elements/Ground  LConnTagsString=a
      settings: SourceProductName=Simscape Electrical
  b : PMIOPort  Side=Right
  B : PMIOPort  Port=2  Side=Left
  connections:
  Ground82/LConn1 -- 2/RConn3 -- 2/RConn1
  Ground83/LConn1 -- 2/LConn3 -- 2/LConn1
  2/RConn2 -- b/RConn1
  2/LConn2 -- B/RConn1
